simulink model "Control"  (R2024a)
settings: Solver=VariableStepAuto  StartTime=0.0  StopTime=500  RelTol=1e-3
undefined symbols (not defined in the file): Aa, Bb, Cc
libraries: slpidlib x1
settings Model: Creator=Preeti Jaiswal  LastModifiedBy=Win

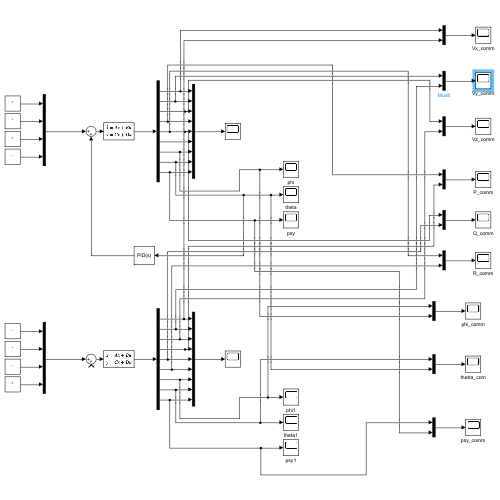
[thumbnail: Simulink's stored preview of the top-level diagram]
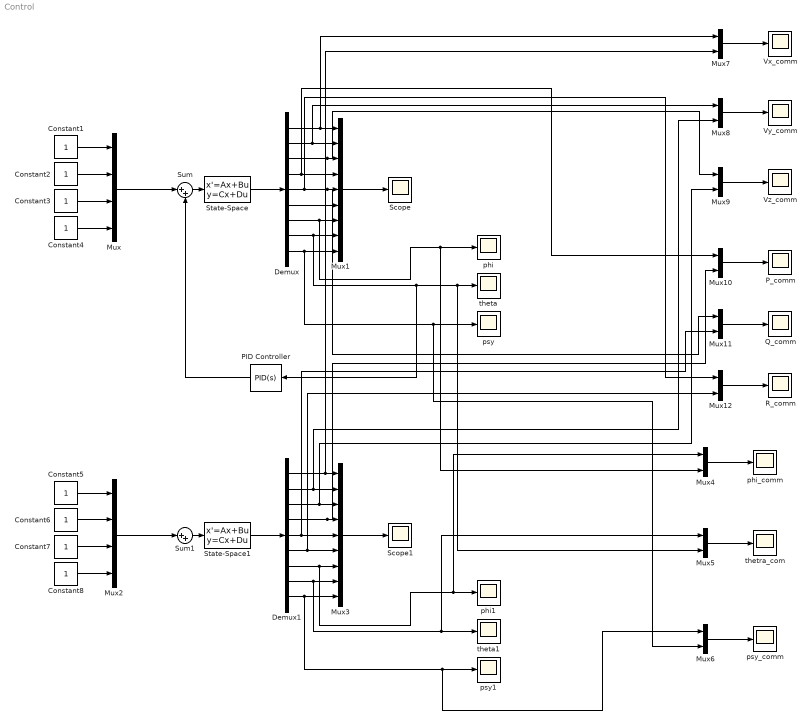
== system Control ==
  Constant{1..8} (8 alike) : Constant
  Demux : Demux  Outputs=9
  Demux1 : Demux  Outputs=9
  Mux : Mux
  Mux1 : Mux  Inputs=9
  Mux{4..12} (9 alike) : Mux  Inputs=2
  Mux2 : Mux
  Mux3 : Mux  Inputs=9
  PID Controller : slpidlib/PID Controller  Controller=PID  Form=Parallel  TimeDomain=Continuous-time  UseExternalTs=off  SampleTime=-1  IntegratorMethod=Forward Euler  FilterMethod=Forward Euler  ControllerParametersSource=internal  P=-1407.5141242506  I=-65.8924616524418  UseKiTs=off  D=-7382.66359610517  UseExternalDerivativeSource=off  N=5.45397025421619  UseFilter=on  TunerSelectOption=Transfer Function Based (PID Tuner App)  InitialConditionSource=internal  InitialConditionForIntegrator=0  InitialConditionForFilter=0  DifferentiatorICPrevScaledInput=0  ExternalReset=none  TrackingMode=off  Kt=1  LimitOutput=off  SatLimitsSource=internal  UpperSaturationLimit=inf  LowerSaturationLimit=-inf  LinearizeAsGain=on  AntiWindupMode=none  Kb=1  LimitIntegrator=off  UpperIntegratorSaturationLimit=inf  LowerIntegratorSaturationLimit=-inf  POutMin=[]  POutMax=[]  IOutMin=[]  IOutMax=[]  DOutMin=[]  DOutMax=[]  NOutMin=[]  NOutMax=[]  SumOutMin=[]  SumOutMax=[]  SaturationOutMin=[]  SaturationOutMax=[]  PParamMin=[]  PParamMax=[]  IParamMin=[]  IParamMax=[]  DParamMin=[]  DParamMax=[]  NParamMin=[]  NParamMax=[]  KbParamMin=[]  KbParamMax=[]  KtParamMin=[]  KtParamMax=[]  KbOutMin=[]  KbOutMax=[]  KtOutMin=[]  KtOutMax=[]  IntegratorOutMin=[]  IntegratorOutMax=[]  FilterOutMin=[]  FilterOutMax=[]  SumI1OutMin=[]  SumI1OutMax=[]  SumI2OutMin=[]  SumI2OutMax=[]  SumI3OutMin=[]  SumI3OutMax=[]  SumI4OutMin=[]  SumI4OutMax=[]  SumDOutMin=[]  SumDOutMax=[]  DifferentiatorOutMin=[]  DifferentiatorOutMax=[]  FilterDiffOutCoefMin=[]  FilterDiffOutCoefMax=[]  ReciprocalOutMin=[]  ReciprocalOutMax=[]  SumDenOutMin=[]  SumDenOutMax=[]  SumNumOutMin=[]  SumNumOutMax=[]  DivideOutMin=[]  DivideOutMax=[]  UdiffTsProdOutMin=[]  UdiffTsProdOutMax=[]  NTsProdOutMin=[]  NTsProdOutMax=[]  UintegralTsProdOutMin=[]  UintegralTsProdOutMax=[]  UngainTsProdOutMin=[]  UngainTsProdOutMax=[]  ClampingZeroOutDataTypeStr=Inherit: Inherit via back propagation  ClampingZeroOutMin=[]  ClampingZeroOutMax=[]  FilterDenConstantOutDataTypeStr=Inherit: Inherit via back propagation  FilterDenConstantOutMin=[]  FilterDenConstantOutMax=[]  PCopyOutDataTypeStr=Inherit: Inherit via back propagation  PCopyOutMin=[]  PCopyOutMax=[]  NCopyOutDataTypeStr=Inherit: Inherit via back propagation  NCopyOutMin=[]  NCopyOutMax=[]  IntegratorContinuousStateAttributes=''  IntegratorStateMustResolveToSignalObject=off  IntegratorRTWStateStorageClass=Auto  FilterContinuousStateAttributes=''  FilterStateMustResolveToSignalObject=off  FilterRTWStateStorageClass=Auto  ParallelPVariant=InternalParameters  IdealPVariant=Disabled  IVariant=InternalParameters  DVariant=InternalParameters  IntegratorVariant=Continuous  SatVariant=Disabled  AWVariant=Passthrough  PCopyVariant=Disabled  TRVariant=Disabled  FdbkBlocksVariant=Forward  IdealPFdbkVariant=Disabled  SatFdbkVariant=Disabled  DerivativeFilterVariant=ContFilter  NVariant=InternalParameters  NCopyVariant=Disabled  FilterICVariant=InternalICsFilter  IntegratorICVariant=InternalICs  ExternalResetVariant=Disabled  TRSumVariant=Passthrough  SumFdbkVariant=Disabled  SumVariant=Sum_PID  TsampFilterVariant=InternalTs  TsampNgainVariant=Passthrough  TsampIntegralVariant=Disabled_SignalSpec  ExternalSaturationOutDataTypeStr=Inherit: Same as second input  DerivativeSourceVariant=ErrorSignal
  P_comm : Scope
  Q_comm : Scope
  R_comm : Scope
  Scope : Scope
  Scope1 : Scope
  State-Space : StateSpace  A=Aa  B=Bb  C=Cc  D=zeros(9, 4)  InitialCondition=0
  State-Space1 : StateSpace  A=Aa  B=Bb  C=Cc  D=zeros(9, 4)  InitialCondition=0
  Sum : Sum  Inputs=|++
  Sum1 : Sum  Inputs=|++
  Vx_comm : Scope
  Vy_comm : Scope
  Vz_comm : Scope
  phi : Scope
  phi1 : Scope
  phi_comm : Scope
  psy : Scope
  psy1 : Scope
  psy_comm : Scope
  theta : Scope
  theta1 : Scope
  thetra_com : Scope
  wires:
  Constant1/1 -> Mux/1
  Constant2/1 -> Mux/2
  Constant3/1 -> Mux/3
  Constant4/1 -> Mux/4
  State-Space/1 -> Demux/1
  Demux/1 -> Mux7/1, Mux1/1
  Demux/2 -> Mux8/1, Mux1/2
  Demux/3 -> Mux9/1, Mux1/3
  Demux/4 -> Mux1/4, Mux10/1
  Demux/5 -> Mux12/1, Mux11/1, Mux1/5
  Demux/6 -> Mux1/6
  Demux/7 -> Mux4/2, phi/1, Mux1/7
  Demux/8 -> PID Controller/1, Mux5/2, theta/1, Mux1/8
  Demux/9 -> Mux6/2, psy/1, Mux1/9
  Mux1/1 -> Scope/1
  Sum/1 -> State-Space/1
  PID Controller/1 -> Sum/2
  Mux/1 -> Sum/1
  Mux2/1 -> Sum1/1
  Demux1/5 -> Mux3/5, Mux11/2
  Demux1/3 -> Mux9/2, Mux3/3
  Demux1/8 -> Mux5/1, theta1/1, Mux3/8
  Sum1/1 -> State-Space1/1
  Demux1/9 -> Mux6/1, psy1/1, Mux3/9
  Demux1/1 -> Mux7/2, Mux3/1
  Constant5/1 -> Mux2/1
  Constant6/1 -> Mux2/2
  Constant8/1 -> Mux2/4
  Mux3/1 -> Scope1/1
  Constant7/1 -> Mux2/3
  Demux1/2 -> Mux8/2, Mux3/2
  Demux1/7 -> Mux4/1, phi1/1, Mux3/7
  Demux1/4 -> Mux10/2, Mux3/4
  Demux1/6 -> Mux3/6, Mux12/2
  State-Space1/1 -> Demux1/1
  Mux4/1 -> phi_comm/1
  Mux5/1 -> thetra_com/1
  Mux6/1 -> psy_comm/1
  Mux9/1 -> Vz_comm/1
  Mux8/1 -> Vy_comm/1
  Mux7/1 -> Vx_comm/1
  Mux12/1 -> R_comm/1
  Mux11/1 -> Q_comm/1
  Mux10/1 -> P_comm/1
